simulink model "Stimulus"  (R2023b)
settings: Solver=VariableStepAuto  StartTime=0.0  StopTime=num_samples/fs  RelTol=1e-3
values from neighbouring files (symbols this model uses):
  fs = 16e6    (= 16000000)    [startup.m]
settings Model: Creator=andre  LastModifiedBy=andre

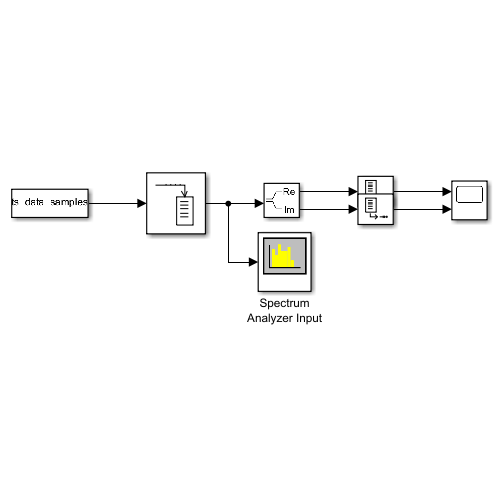
[thumbnail: Simulink's stored preview of the top-level diagram]
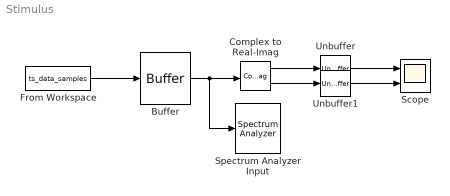
== system Stimulus ==
  Buffer : Buffer  N=2048  OutputFrames=off
  Complex to Real-Imag : ComplexToRealImag
  From Workspace : FromWorkspace  VariableName=ts_data_samples  SampleTime=1/fs
  Scope : Scope  NumInputPorts=2
  Spectrum Analyzer Input : SpectrumAnalyzer  WindowPosition=[1921.000000,-319.000000,1920.000000,1017.000000,]  Visible=on  ScopeFrameLocation=window  ViewType=Spectrum and spectrogram  Span=128000000  StartFrequency=-64000000  StopFrequency=64000000  TimeSpanSource=Property  TimeSpan=0.110592  YLimits=[-15.6057143,7.09813491]  ColorLimits=[-15.6057143,7.09813491]  SelectedToolstripTab=spectrumAnalyzerToolstrip.spectrogramTab
  Unbuffer : Unbuffer
  Unbuffer1 : Unbuffer
  wires:
  From Workspace/1 -> Buffer/1
  Buffer/1 -> Spectrum Analyzer Input/1, Complex to Real-Imag/1
  Complex to Real-Imag/1 -> Unbuffer/1
  Complex to Real-Imag/2 -> Unbuffer1/1
  Unbuffer/1 -> Scope/1
  Unbuffer1/1 -> Scope/2
